simulink model "bacteriaPopulation"  (R2017a)
settings: Solver=VariableStepAuto  StartTime=0.0  StopTime=10.0  RelTol=1e-3
undefined symbols (not defined in the file): contractAfterSimulation, ContractAssumeBlock, contractBeforeSimulation, ContractBlock, ContractEnsureBlock, ContractGuaranteeBlock, ContractModeBlock, ContractRequireBlock, ContractValidatorBlock
libraries: Kind x15, simulink x4
settings Model: Creator=mahgoubyahia  LastModifiedBy=mahgoubyahia

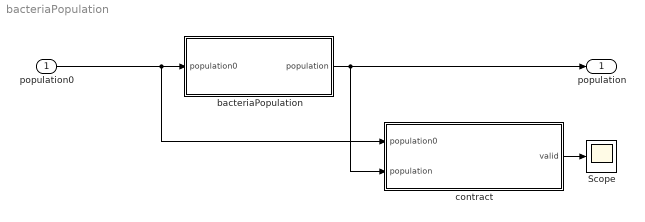
== system bacteriaPopulation ==
  population0 : Inport
  Scope : Scope
  bacteriaPopulation : Subsystem
  contract : Subsystem  mask{ContractBlockType=ContractBlock}
      mask init:
      | set_param(gcb, 'LinkStatus', 'none');
      mask DialogControl DescTextVar Prompt: Contract block
      mask Display:
      | text(0.5, 0.5, '{\bf\fontsize{20}Contract}', 'hor', 'center', 'texmode','on');
      | blocks = find_system(gcb, 'LookUnderMasks','all', 'SearchDepth',1,'BlockType','Inport');
      | for i = 1 : length(blocks)
      |     blockName = get_param(blocks(i), 'Name');
      |     [path, blockName] = fileparts(char(blockName));
      |     port_label('input', i, blockName);
      | end
      | 
      | blocks = find_system(gcb, 'LookUnderMasks','all', 'SearchDepth',1,'BlockType','Outport');
      | for i = 1 : length(blocks)
      |     blockName = get_param(blocks(i), 'Name');
      |     [path, blockName] = fileparts(char(blockName));
      |     port_label('output', i, blockName);
      | end
  population : Outport
  wires:
  population0/1 -> bacteriaPopulation/1(population0), contract/1(population0)
  contract/1(valid) -> Scope/1
  bacteriaPopulation/1(population) -> contract/2(population), population/1

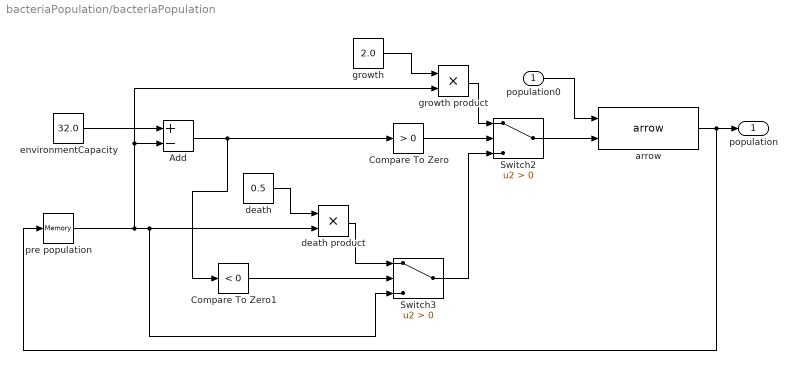
== system bacteriaPopulation/bacteriaPopulation ==
  population0 : Inport
  Add : Sum  Inputs=+-
  Compare To Zero : simulink/Logic and Bit Operations/Compare To Zero  relop=>  OutDataTypeStr=boolean
  Compare To Zero1 : simulink/Logic and Bit Operations/Compare To Zero  relop=<  OutDataTypeStr=boolean
  Switch2 : Switch  Criteria=u2 > Threshold
  Switch3 : Switch  Criteria=u2 > Threshold
  arrow : Kind/arrow  LustreOperatorBlock=ArrowOperator
      settings: SourceProductName=Kind lib
  death : Constant  Value=0.5  OutDataTypeStr=double
  death product : Product
  environmentCapacity : Constant  Value=32.0  OutDataTypeStr=double
  growth : Constant  Value=2.0  OutDataTypeStr=double
  growth product : Product
  pre population : Memory
  population : Outport
  wires:
  growth/1 -> growth product/1
  Add/1 -> Compare To Zero1/1, Compare To Zero/1
  growth product/1 -> Switch2/1
  Compare To Zero1/1 -> Switch3/2
  environmentCapacity/1 -> Add/1
  Compare To Zero/1 -> Switch2/2
  Switch3/1 -> Switch2/3
  Switch2/1 -> arrow/2
  pre population/1 -> Switch3/3, death product/2, Add/2, growth product/2
  population0/1 -> arrow/1
  death/1 -> death product/1
  death product/1 -> Switch3/1
  arrow/1 -> pre population/1, population/1

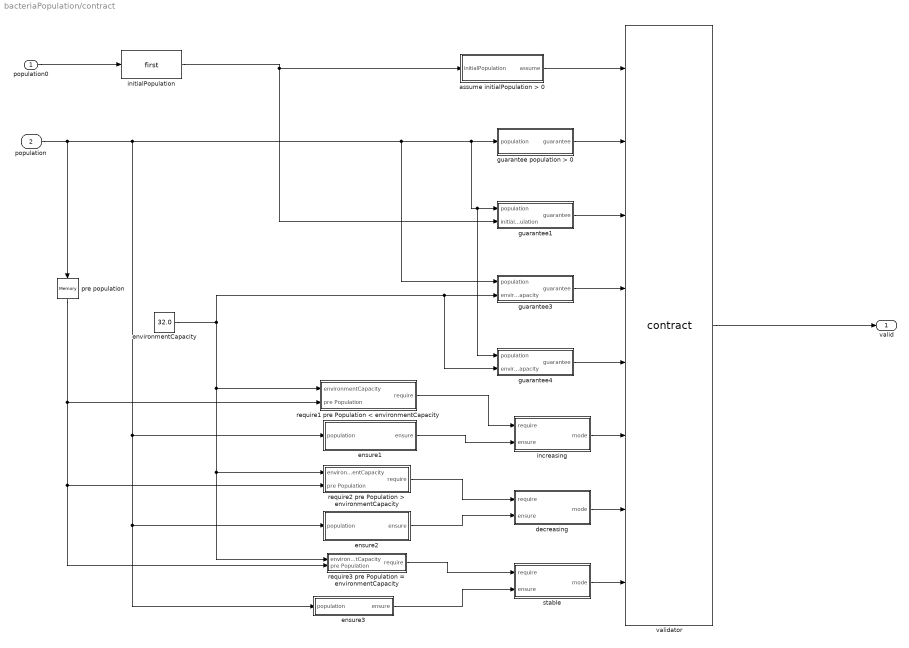
== system bacteriaPopulation/contract ==
  population0 : Inport
  population : Inport  Port=2
  assume initialPopulation > 0 : Subsystem  mask{ContractBlockType=ContractAssumeBlock}
      mask init:
      | set_param(gcb, 'LinkStatus', 'none');
      mask DialogControl DescTextVar Prompt: Assume block
  decreasing : Subsystem  mask{ContractBlockType=ContractModeBlock}
      mask init:
      | set_param(gcb, 'LinkStatus', 'none');
      mask DialogControl DescTextVar Prompt: Mode block
  ensure1 : Subsystem  mask{ContractBlockType=ContractEnsureBlock}
      mask init:
      | set_param(gcb, 'LinkStatus', 'none');
      mask DialogControl DescTextVar Prompt: Ensure block
  ensure2 : Subsystem  mask{ContractBlockType=ContractEnsureBlock}
      mask init:
      | set_param(gcb, 'LinkStatus', 'none');
      mask DialogControl DescTextVar Prompt: Ensure block
  ensure3 : Subsystem  mask{ContractBlockType=ContractEnsureBlock}
      mask init:
      | set_param(gcb, 'LinkStatus', 'none');
      mask DialogControl DescTextVar Prompt: Ensure block
  environmentCapacity : Constant  Value=32.0  OutDataTypeStr=double
  guarantee population > 0 : Subsystem  mask{ContractBlockType=ContractGuaranteeBlock}
      mask init:
      | set_param(gcb, 'LinkStatus', 'none');
      mask DialogControl DescTextVar Prompt: Guarantee block
  guarantee1 : Subsystem  mask{ContractBlockType=ContractGuaranteeBlock}
      mask init:
      | set_param(gcb, 'LinkStatus', 'none');
      mask DialogControl DescTextVar Prompt: Guarantee block
  guarantee3 : Subsystem  mask{ContractBlockType=ContractGuaranteeBlock}
      mask init:
      | set_param(gcb, 'LinkStatus', 'none');
      mask DialogControl DescTextVar Prompt: Guarantee block
  guarantee4 : Subsystem  mask{ContractBlockType=ContractGuaranteeBlock}
      mask init:
      | set_param(gcb, 'LinkStatus', 'none');
      mask DialogControl DescTextVar Prompt: Guarantee block
  increasing : Subsystem  mask{ContractBlockType=ContractModeBlock}
      mask init:
      | set_param(gcb, 'LinkStatus', 'none');
      mask DialogControl DescTextVar Prompt: Mode block
  initialPopulation : Kind/first  SystemSampleTime=-1
      settings: SourceProductName=Kind lib
  pre population : Memory
  require1 pre Population < environmentCapacity : Subsystem  mask{ContractBlockType=ContractRequireBlock}
      mask init:
      | set_param(gcb, 'LinkStatus', 'none');
      mask DialogControl DescTextVar Prompt: Require block
  require2 pre Population > environmentCapacity : Subsystem  mask{ContractBlockType=ContractRequireBlock}
      mask init:
      | set_param(gcb, 'LinkStatus', 'none');
      mask DialogControl DescTextVar Prompt: Require block
  require3 pre Population = environmentCapacity : Subsystem  mask{ContractBlockType=ContractRequireBlock}
      mask init:
      | set_param(gcb, 'LinkStatus', 'none');
      mask DialogControl DescTextVar Prompt: Require block
  stable : Subsystem  mask{ContractBlockType=ContractModeBlock}
      mask init:
      | set_param(gcb, 'LinkStatus', 'none');
      mask DialogControl DescTextVar Prompt: Mode block
  validator : M-S-Function  LoadFcn=|  InitFcn=contractBeforeSimulation();  StopFcn=contractAfterSimulation();  FunctionName=contract  mask{assumePorts=1, guaranteePorts=4, modePorts=3, ContractBlockType=ContractValidatorBlock, createInportsCheckbox=off, createEnsureRequireCheckbox=off}
      | values = get_param(gcb,'MaskValues');
      | ContractValidatorBlock.block = gcb;
      | ContractValidatorBlock.assumePorts = ... 
      |     str2num(char(values(1)));
      | ContractValidatorBlock.guaranteePorts = ...
      |     str2num(char(values(2)));
      | ContractValidatorBlock.modeBlocksPorts = ...
      |     str2num(char(values(3)));
      | 
      | ContractValidatorBlock.portHandles = ...
      |     get_param(ContractValidatorBlock.block, 'PortHandles');
      | ContractValidatorBlock.portConnectivity = ...
      |     get_param(ContractValidatorBlock.block, 'PortConnectivity');
      mask prompts: assumePorts "Assume ports     :"; guaranteePorts "Guarantee ports :"; modePorts "Mode ports        :"; createInportsCheckbox "Create inports and connect them automatically"; createEnsureRequireCheckbox "Create ensure and require blocks for mode blocks"
      mask init:
      | set_param(gcb,'LinkStatus','none');
      | contract_callback('inputs_callback',gcb);
      mask DialogControl DescTextVar Prompt: The validator block implements the following logic: <br> <br> <b>Sofar</b>(assume<sub>1</sub> <b>&#8743;</b> assume<sub>2</sub> <b>&#8743;</b> ... assume<sub>k</sub>) <b>&rarr;</b> (guarantee<sub>1</sub> <b>&#8743;</b> guarantee<sub>2</sub> <b>&#8743;</b> ... guarantee<sub>m</sub> <b>&#8743;</b>  mode<sub>1</sub> <b>&#8743;</b> mode<sub>2</sub> <b>&#8743;</b> ... <b>&#8743;</b> mode<sub>n</sub> )<br> where mode<sub>i</sub> = require<sub>i</sub> <b>&rarr;</b> ensure<sub>i</sub>
      mask Display:
      | port_label('input',1,'assume')
      | port_label('input',2,'guarantee')
      | port_label('input',3,'guarantee')
      | port_label('input',4,'guarantee')
      | port_label('input',5,'guarantee')
      | port_label('input',6,'mode')
      | port_label('input',7,'mode')
      | port_label('input',8,'mode')
      | port_label('output',1,'valid')
  valid : Outport
  wires:
  validator/1 -> valid/1
  population0/1 -> initialPopulation/1
  population/1 -> pre population/1, ensure1/1(population), ensure3/1(population), ensure2/1(population), guarantee4/1(population), guarantee1/1(population), guarantee population > 0/1(population), guarantee3/1(population)
  require1 pre Population < environmentCapacity/1(require) -> increasing/1(require)
  ensure1/1(ensure) -> increasing/2(ensure)
  require2 pre Population > environmentCapacity/1(require) -> decreasing/1(require)
  ensure2/1(ensure) -> decreasing/2(ensure)
  require3 pre Population = environmentCapacity/1(require) -> stable/1(require)
  ensure3/1(ensure) -> stable/2(ensure)
  environmentCapacity/1 -> require3 pre Population = environmentCapacity/1(environmentCapacity), require2 pre Population > environmentCapacity/1(environmentCapacity), require1 pre Population < environmentCapacity/1(environmentCapacity), guarantee4/2(environmentCapacity), guarantee3/2(environmentCapacity)
  initialPopulation/1 -> assume initialPopulation > 0/1(initialPopulation), guarantee1/2(initialPopulation)
  assume initialPopulation > 0/1(assume) -> validator/1
  guarantee population > 0/1(guarantee) -> validator/2
  guarantee1/1(guarantee) -> validator/3
  guarantee3/1(guarantee) -> validator/4
  increasing/1(mode) -> validator/6
  decreasing/1(mode) -> validator/7
  stable/1(mode) -> validator/8
  guarantee4/1(guarantee) -> validator/5
  pre population/1 -> require1 pre Population < environmentCapacity/2(pre Population), require2 pre Population > environmentCapacity/2(pre Population), require3 pre Population = environmentCapacity/2(pre Population)

== system bacteriaPopulation/contract/assume initialPopulation > 0 ==
  initialPopulation : Inport
  Compare To Zero : simulink/Logic and Bit Operations/Compare To Zero  relop=>  OutDataTypeStr=boolean
  assume : Outport  OutDataTypeStr=boolean
  wires:
  initialPopulation/1 -> Compare To Zero/1
  Compare To Zero/1 -> assume/1

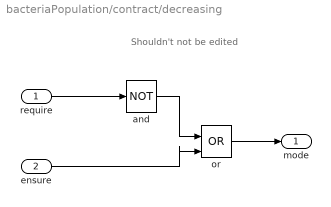
== system bacteriaPopulation/contract/decreasing ==
  note: Shouldn't not be edited
  require : Inport  OutDataTypeStr=boolean
  ensure : Inport  Port=2  OutDataTypeStr=boolean
  and : Logic  Operator=NOT  IconShape=distinctive  AllPortsSameDT=off  OutDataTypeStr=boolean
  or : Logic  Operator=OR  IconShape=distinctive  AllPortsSameDT=off  OutDataTypeStr=boolean
  mode : Outport
  wires:
  require/1 -> and/1
  ensure/1 -> or/2
  and/1 -> or/1
  or/1 -> mode/1

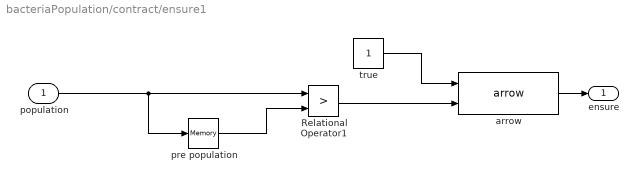
== system bacteriaPopulation/contract/ensure1 ==
  population : Inport
  Relational Operator1 : RelationalOperator  Operator=>  OutDataTypeStr=boolean  RndMeth=Simplest
  arrow : Kind/arrow  LustreOperatorBlock=ArrowOperator
      settings: SourceProductName=Kind lib
  pre population : Memory
  true : Constant  OutDataTypeStr=boolean
  ensure : Outport  OutDataTypeStr=boolean
  wires:
  pre population/1 -> Relational Operator1/2
  true/1 -> arrow/1
  Relational Operator1/1 -> arrow/2
  arrow/1 -> ensure/1
  population/1 -> pre population/1, Relational Operator1/1

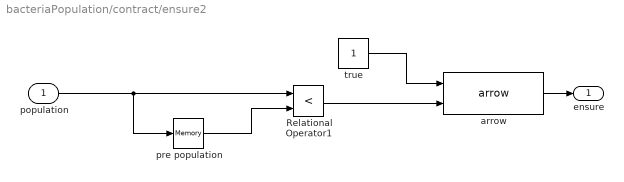
== system bacteriaPopulation/contract/ensure2 ==
  population : Inport
  Relational Operator1 : RelationalOperator  Operator=<  OutDataTypeStr=boolean  RndMeth=Simplest
  arrow : Kind/arrow  LustreOperatorBlock=ArrowOperator
      settings: SourceProductName=Kind lib
  pre population : Memory
  true : Constant  OutDataTypeStr=boolean
  ensure : Outport  OutDataTypeStr=boolean
  wires:
  pre population/1 -> Relational Operator1/2
  true/1 -> arrow/1
  Relational Operator1/1 -> arrow/2
  arrow/1 -> ensure/1
  population/1 -> pre population/1, Relational Operator1/1

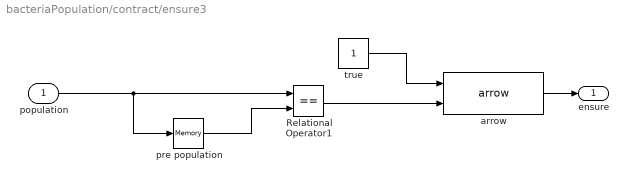
== system bacteriaPopulation/contract/ensure3 ==
  population : Inport
  Relational Operator1 : RelationalOperator  Operator===  OutDataTypeStr=boolean  RndMeth=Simplest
  arrow : Kind/arrow  LustreOperatorBlock=ArrowOperator
      settings: SourceProductName=Kind lib
  pre population : Memory
  true : Constant  OutDataTypeStr=boolean
  ensure : Outport  OutDataTypeStr=boolean
  wires:
  Relational Operator1/1 -> arrow/2
  true/1 -> arrow/1
  arrow/1 -> ensure/1
  population/1 -> pre population/1, Relational Operator1/1
  pre population/1 -> Relational Operator1/2

== system bacteriaPopulation/contract/guarantee population > 0 ==
  population : Inport
  Compare To Zero1 : simulink/Logic and Bit Operations/Compare To Zero  relop=>  OutDataTypeStr=boolean
  guarantee : Outport  OutDataTypeStr=boolean
  wires:
  population/1 -> Compare To Zero1/1
  Compare To Zero1/1 -> guarantee/1

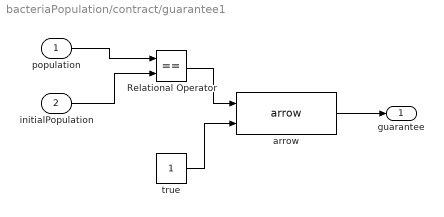
== system bacteriaPopulation/contract/guarantee1 ==
  population : Inport
  initialPopulation : Inport  Port=2
  Relational Operator : RelationalOperator  Operator===  OutDataTypeStr=boolean  RndMeth=Simplest
  arrow : Kind/arrow  LustreOperatorBlock=ArrowOperator
      settings: SourceProductName=Kind lib
  true : Constant  OutDataTypeStr=boolean
  guarantee : Outport  OutDataTypeStr=boolean
  wires:
  arrow/1 -> guarantee/1
  true/1 -> arrow/2
  population/1 -> Relational Operator/1
  initialPopulation/1 -> Relational Operator/2
  Relational Operator/1 -> arrow/1

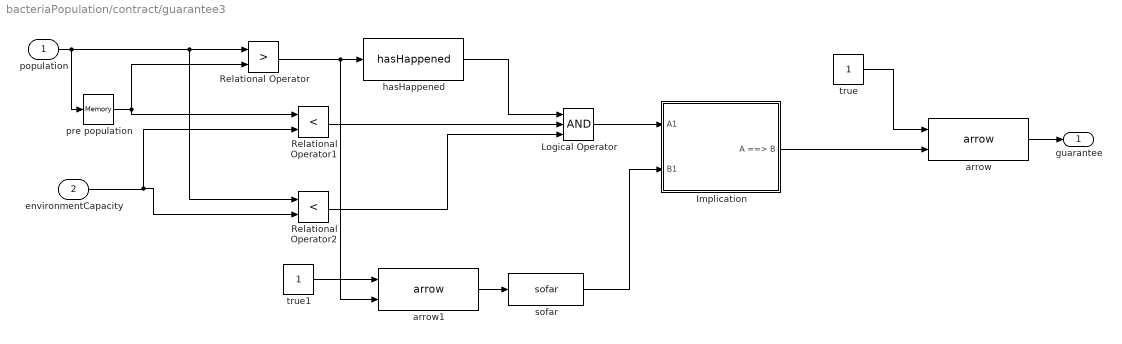
== system bacteriaPopulation/contract/guarantee3 ==
  population : Inport
  environmentCapacity : Inport  Port=2
  Implication : Subsystem  mask(CoCoSim-Implies){}
      mask help: CoCoSim block for Logical Implication
      mask Display: disp(' ')
  Logical Operator : Logic  Inputs=3  AllPortsSameDT=off  OutDataTypeStr=boolean
  Relational Operator : RelationalOperator  Operator=>  OutDataTypeStr=boolean  RndMeth=Simplest
  Relational Operator1 : RelationalOperator  Operator=<  OutDataTypeStr=boolean  RndMeth=Simplest
  Relational Operator2 : RelationalOperator  Operator=<  OutDataTypeStr=boolean  RndMeth=Simplest
  arrow : Kind/arrow  LustreOperatorBlock=ArrowOperator
      settings: SourceProductName=Kind lib
  arrow1 : Kind/arrow  LustreOperatorBlock=ArrowOperator
      settings: SourceProductName=Kind lib
  hasHappened : Kind/hasHappened  SystemSampleTime=-1
      settings: SourceProductName=Kind lib
  pre population : Memory
  sofar : Kind/sofar  SystemSampleTime=-1
      settings: SourceProductName=Kind lib
  true : Constant  OutDataTypeStr=boolean
  true1 : Constant  OutDataTypeStr=boolean
  guarantee : Outport  OutDataTypeStr=boolean
  wires:
  population/1 -> pre population/1, Relational Operator2/1, Relational Operator/1
  pre population/1 -> Relational Operator1/1, Relational Operator/2
  Relational Operator/1 -> arrow1/2, hasHappened/1
  hasHappened/1 -> Logical Operator/1
  environmentCapacity/1 -> Relational Operator2/2, Relational Operator1/2
  arrow/1 -> guarantee/1
  Relational Operator1/1 -> Logical Operator/2
  Relational Operator2/1 -> Logical Operator/3
  true/1 -> arrow/1
  true1/1 -> arrow1/1
  Logical Operator/1 -> Implication/1(A1)
  sofar/1 -> Implication/2(B1)
  arrow1/1 -> sofar/1
  Implication/1(A ==> B) -> arrow/2

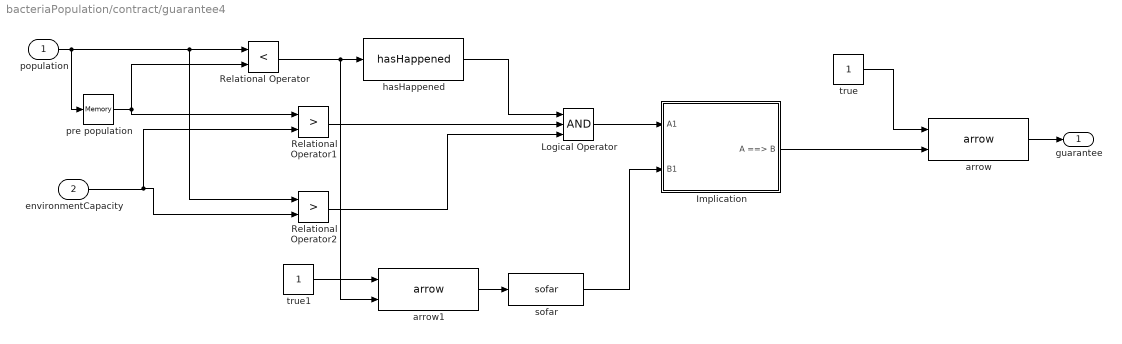
== system bacteriaPopulation/contract/guarantee4 ==
  population : Inport
  environmentCapacity : Inport  Port=2
  Implication : Subsystem  mask(CoCoSim-Implies){}
      mask help: CoCoSim block for Logical Implication
      mask Display: disp(' ')
  Logical Operator : Logic  Inputs=3  AllPortsSameDT=off  OutDataTypeStr=boolean
  Relational Operator : RelationalOperator  Operator=<  OutDataTypeStr=boolean  RndMeth=Simplest
  Relational Operator1 : RelationalOperator  Operator=>  OutDataTypeStr=boolean  RndMeth=Simplest
  Relational Operator2 : RelationalOperator  Operator=>  OutDataTypeStr=boolean  RndMeth=Simplest
  arrow : Kind/arrow  LustreOperatorBlock=ArrowOperator
      settings: SourceProductName=Kind lib
  arrow1 : Kind/arrow  LustreOperatorBlock=ArrowOperator
      settings: SourceProductName=Kind lib
  hasHappened : Kind/hasHappened  SystemSampleTime=-1
      settings: SourceProductName=Kind lib
  pre population : Memory
  sofar : Kind/sofar  SystemSampleTime=-1
      settings: SourceProductName=Kind lib
  true : Constant  OutDataTypeStr=boolean
  true1 : Constant  OutDataTypeStr=boolean
  guarantee : Outport  OutDataTypeStr=boolean
  wires:
  Relational Operator2/1 -> Logical Operator/3
  Implication/1(A ==> B) -> arrow/2
  true/1 -> arrow/1
  environmentCapacity/1 -> Relational Operator2/2, Relational Operator1/2
  sofar/1 -> Implication/2(B1)
  Relational Operator/1 -> arrow1/2, hasHappened/1
  arrow1/1 -> sofar/1
  population/1 -> pre population/1, Relational Operator2/1, Relational Operator/1
  pre population/1 -> Relational Operator1/1, Relational Operator/2
  arrow/1 -> guarantee/1
  Relational Operator1/1 -> Logical Operator/2
  Logical Operator/1 -> Implication/1(A1)
  true1/1 -> arrow1/1
  hasHappened/1 -> Logical Operator/1

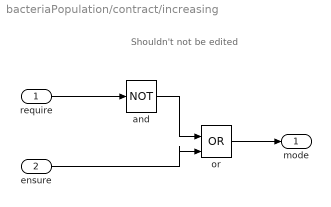
== system bacteriaPopulation/contract/increasing ==
  note: Shouldn't not be edited
  require : Inport  OutDataTypeStr=boolean
  ensure : Inport  Port=2  OutDataTypeStr=boolean
  and : Logic  Operator=NOT  IconShape=distinctive  AllPortsSameDT=off  OutDataTypeStr=boolean
  or : Logic  Operator=OR  IconShape=distinctive  AllPortsSameDT=off  OutDataTypeStr=boolean
  mode : Outport
  wires:
  require/1 -> and/1
  ensure/1 -> or/2
  and/1 -> or/1
  or/1 -> mode/1

== system bacteriaPopulation/contract/require1 pre Population < environmentCapacity ==
  environmentCapacity : Inport
  pre Population : Inport  Port=2
  Relational Operator : RelationalOperator  Operator=<  OutDataTypeStr=boolean  RndMeth=Simplest
  require : Outport  OutDataTypeStr=boolean
  wires:
  pre Population/1 -> Relational Operator/1
  environmentCapacity/1 -> Relational Operator/2
  Relational Operator/1 -> require/1

== system bacteriaPopulation/contract/require2 pre Population > environmentCapacity ==
  environmentCapacity : Inport
  pre Population : Inport  Port=2
  Relational Operator : RelationalOperator  Operator=>  OutDataTypeStr=boolean  RndMeth=Simplest
  require : Outport  OutDataTypeStr=boolean
  wires:
  pre Population/1 -> Relational Operator/1
  Relational Operator/1 -> require/1
  environmentCapacity/1 -> Relational Operator/2

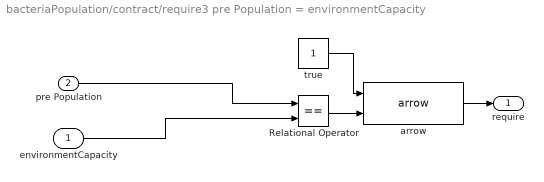
== system bacteriaPopulation/contract/require3 pre Population = environmentCapacity ==
  environmentCapacity : Inport
  pre Population : Inport  Port=2
  Relational Operator : RelationalOperator  Operator===  OutDataTypeStr=boolean  RndMeth=Simplest
  arrow : Kind/arrow  LustreOperatorBlock=ArrowOperator
      settings: SourceProductName=Kind lib
  true : Constant  OutDataTypeStr=boolean
  require : Outport  OutDataTypeStr=boolean
  wires:
  environmentCapacity/1 -> Relational Operator/2
  pre Population/1 -> Relational Operator/1
  true/1 -> arrow/1
  Relational Operator/1 -> arrow/2
  arrow/1 -> require/1

== system bacteriaPopulation/contract/stable ==
  note: Shouldn't not be edited
  require : Inport  OutDataTypeStr=boolean
  ensure : Inport  Port=2  OutDataTypeStr=boolean
  and : Logic  Operator=NOT  IconShape=distinctive  AllPortsSameDT=off  OutDataTypeStr=boolean
  or : Logic  Operator=OR  IconShape=distinctive  AllPortsSameDT=off  OutDataTypeStr=boolean
  mode : Outport
  wires:
  require/1 -> and/1
  ensure/1 -> or/2
  and/1 -> or/1
  or/1 -> mode/1

== system bacteriaPopulation/contract/guarantee3/Implication ==
  A1 : Inport
  B1 : Inport  Port=2
  Logical Operator : Logic  Operator=OR  AllPortsSameDT=off  OutDataTypeStr=boolean
  Logical Operator1 : Logic  Operator=NOT  AllPortsSameDT=off  OutDataTypeStr=boolean
  A ==> B : Outport
  wires:
  A1/1 -> Logical Operator1/1
  Logical Operator1/1 -> Logical Operator/1
  B1/1 -> Logical Operator/2
  Logical Operator/1 -> A ==> B/1

== system bacteriaPopulation/contract/guarantee4/Implication ==
  A1 : Inport
  B1 : Inport  Port=2
  Logical Operator : Logic  Operator=OR  AllPortsSameDT=off  OutDataTypeStr=boolean
  Logical Operator1 : Logic  Operator=NOT  AllPortsSameDT=off  OutDataTypeStr=boolean
  A ==> B : Outport
  wires:
  A1/1 -> Logical Operator1/1
  Logical Operator1/1 -> Logical Operator/1
  B1/1 -> Logical Operator/2
  Logical Operator/1 -> A ==> B/1
